simulink model "G_2"  (R2019a)
settings: Solver=VariableStepAuto  StartTime=0.0  StopTime=40  RelTol=1e-3
values from neighbouring files (symbols this model uses):
  A = sys_d.a    [ss2dt.m]    (also in vars.m = [[ 0.      0.      1.      0.    ])
  B = sys_d.b    [ss2dt.m]    (also in vars.m = [[0.        ])
  C = sys_d.c    [ss2dt.m]    (also in vars.m = [[1. 0. 0. 0.])
  K = [[ -2.00366979 199.78340569  -6.64587178  52.07504646]]    [vars.m]
  L = [[ 2.45    0.15  ] ... (first row only)    [vars.m]
libraries: commchan3 x1
settings Model: Creator=Artem  LastModifiedBy=Artem

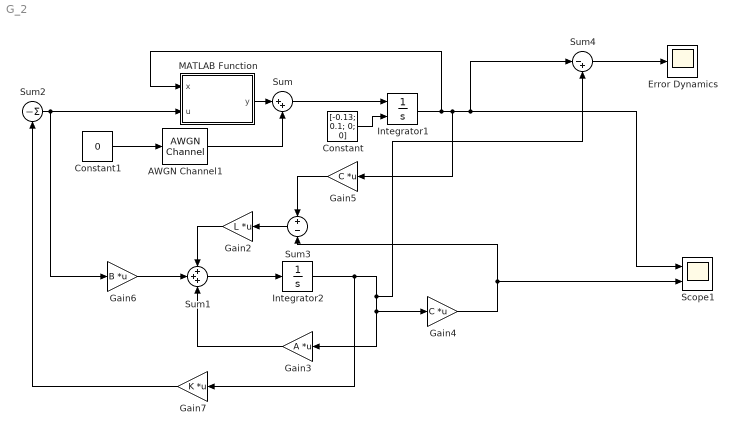
== system G_2 ==
  AWGN Channel1 : commchan3/AWGN Channel  InputProcessing=Columns as channels (frame based)  seed=2  noiseMode=Variance from mask  EbNodB=10  EsNodB=10  SNRdB=10  bitsPerSym=1  Ps=1  Tsym=1  variance=0.0001
      settings: SourceProductName=Communications Toolbox
  Constant : Constant  Value=[-0.13; 0.1; 0; 0]
  Constant1 : Constant  Value=0
  Error Dynamics : Scope
  Gain2 : Gain  Gain=L  Multiplication=Matrix(K*u)
  Gain3 : Gain  Gain=A  Multiplication=Matrix(K*u)
  Gain4 : Gain  Gain=C  Multiplication=Matrix(K*u)
  Gain5 : Gain  Gain=C  Multiplication=Matrix(K*u)
  Gain6 : Gain  Gain=B  Multiplication=Matrix(K*u)
  Gain7 : Gain  Gain=K  Multiplication=Matrix(K*u)
  Integrator1 : Integrator  InitialConditionSource=external
  Integrator2 : Integrator
  MATLAB Function : MATLAB Function  TreatAsAtomicUnit=on
  Scope1 : Scope  NumInputPorts=2
  Sum : Sum  Inputs=|++
  Sum1 : Sum  Inputs=+++
  Sum2 : Sum  Inputs=||-
  Sum3 : Sum  Inputs=+-
  Sum4 : Sum  Inputs=|-+
  wires:
  Integrator1/1 -> MATLAB Function/1(x), Gain5/1, Scope1/1, Sum4/1
  Integrator2/1 -> Gain7/1, Sum4/2, Gain4/1, Gain3/1
  Sum2/1 -> MATLAB Function/2(u), Gain6/1
  Gain2/1 -> Sum1/1
  Sum1/1 -> Integrator2/1
  Gain4/1 -> Scope1/2, Sum3/2
  Gain6/1 -> Sum1/2
  Gain3/1 -> Sum1/3
  Gain7/1 -> Sum2/1
  Constant1/1 -> AWGN Channel1/1
  Sum3/1 -> Gain2/1
  Gain5/1 -> Sum3/1
  Constant/1 -> Integrator1/2
  Sum4/1 -> Error Dynamics/1
  MATLAB Function/1(y) -> Sum/1
  AWGN Channel1/1 -> Sum/2
  Sum/1 -> Integrator1/1

== matlab function G_2/MATLAB Function ==
  data: x input; u input; y output
function y = fcn(x,u)
g = 9.81;
m = 4.4;
M = 7.5;
l = 1.2;


x2 = @(theta,theta_, F) (m * sin(theta) * (g * cos(theta)  - l * theta_ ^ 2) + F) / (M + m * sin(theta) ^ 2);   %(- l*m*sin(theta)*theta_^2 + F + cos(theta)*g*m*sin(theta))/(- m*cos(theta)^2 + M + m);
theta2 = @(theta,theta_, F) ((g * (M+m)-l*m*cos(theta)*theta_^2 )* sin(theta) + F * cos(theta))/ (l * (M + m * sin(theta)^2)); %-(- l*m*sin(theta)*theta_^2 + F + (g*sin(theta)*(M + m))/cos(theta))/(l*cos(theta)*m - (l*(M + m))/cos(theta));

y = [  x(3);
       x(4);
       x2(x(2),x(4),u);
       theta2(x(2),x(4),u)];
